simulink model "SOC_Estimation_2RC"  (R2022a)
settings: Solver=VariableStepAuto  StartTime=0.0  StopTime=3600  RelTol=1e-3
libraries: fl_lib x9, nesl_utility x4, simulink x2
settings Model: Creator=10109  LastModifiedBy=10109

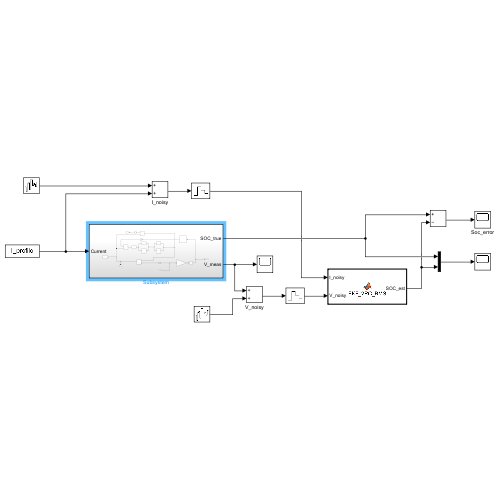
[thumbnail: Simulink's stored preview of the top-level diagram]
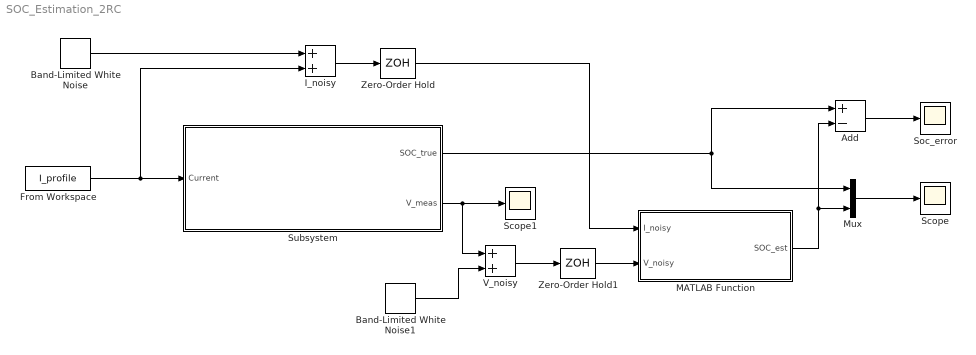
== system SOC_Estimation_2RC ==
  Add : Sum  Inputs=+-
  Band-Limited White Noise : simulink/Sources/Band-Limited White Noise  Cov=[4e-4]  Ts=1  seed=[2334]
  Band-Limited White Noise1 : simulink/Sources/Band-Limited White Noise  Cov=[1e-4]  Ts=1  seed=[2335]
  From Workspace : FromWorkspace  VariableName=I_profile
  I_noisy : Sum
  MATLAB Function : MATLAB Function  TreatAsAtomicUnit=on
  Mux : Mux  Inputs=2
  Scope : Scope
  Scope1 : Scope
  Soc_error : Scope
  Subsystem : Subsystem
  V_noisy : Sum
  Zero-Order Hold : ZeroOrderHold
  Zero-Order Hold1 : ZeroOrderHold
  wires:
  Subsystem/2(V_meas) -> Scope1/1, V_noisy/1
  Band-Limited White Noise1/1 -> V_noisy/2
  From Workspace/1 -> Subsystem/1(Current), I_noisy/2
  Band-Limited White Noise/1 -> I_noisy/1
  Subsystem/1(SOC_true) -> Add/1, Mux/1
  MATLAB Function/1(SOC_est) -> Add/2, Mux/2
  Zero-Order Hold1/1 -> MATLAB Function/2(V_noisy)
  I_noisy/1 -> Zero-Order Hold/1
  Zero-Order Hold/1 -> MATLAB Function/1(I_noisy)
  V_noisy/1 -> Zero-Order Hold1/1
  Mux/1 -> Scope/1
  Add/1 -> Soc_error/1

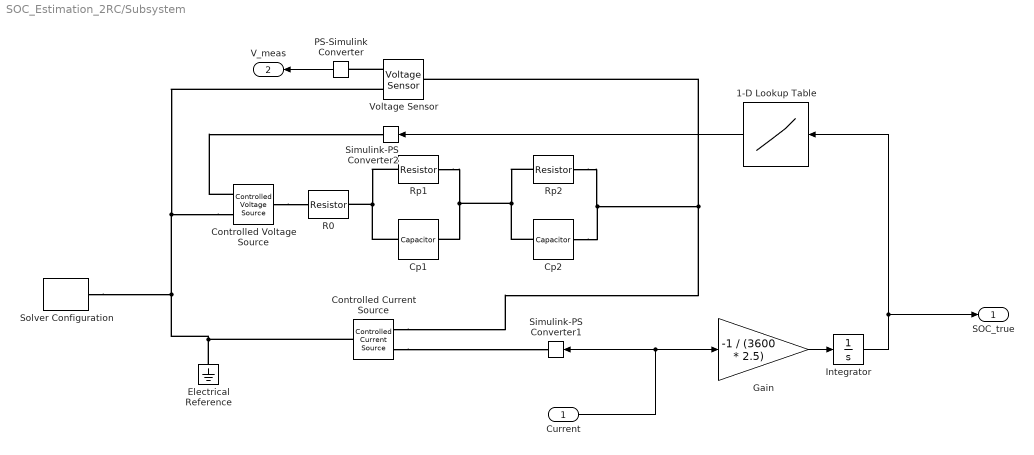
== system SOC_Estimation_2RC/Subsystem ==
  Current : Inport
  1-D Lookup Table : Lookup_n-D  NumberOfTableDimensions=1  BreakpointsForDimension1=[0, 0.1, 0.2, 0.3, 0.4, 0.5, 0.6, 0.7, 0.8, 0.9, 1.0]  Table=[3.00, 3.45, 3.55, 3.62, 3.68, 3.74, 3.82, 3.92, 4.02, 4.12, 4.20]  ExtrapMethod=Clip  UseLastTableValue=on  InternalRulePriority=Speed  RndMeth=Simplest
  Controlled Current Source : fl_lib/Electrical/Electrical Sources/Controlled Current Source
      settings: SourceProductBaseCode=PW,SS,VE
  Controlled Voltage Source : fl_lib/Electrical/Electrical Sources/Controlled Voltage Source
      settings: SourceProductBaseCode=PW,SS,VE
  Cp1 : fl_lib/Electrical/Electrical Elements/Capacitor  c=250 F  r=1e-6 Ohm  g=0 1/Ohm  i_specify=off  i_priority=None  i=0 A  i_nominal_specify=off  i_nominal_unit=A  i_nominal_value=1  v_specify=off  v_priority=None  v=0 V  v_nominal_specify=off  v_nominal_unit=V  v_nominal_value=1  vc_specify=off  vc_priority=High  vc=0 V  vc_nominal_specify=off  vc_nominal_unit=V  vc_nominal_value=1
      settings: SourceProductBaseCode=PW,SS,VE
  Cp2 : fl_lib/Electrical/Electrical Elements/Capacitor  c=1200 F  r=1e-6 Ohm  g=0 1/Ohm  i_specify=off  i_priority=None  i=0 A  i_nominal_specify=off  i_nominal_unit=A  i_nominal_value=1  v_specify=off  v_priority=None  v=0 V  v_nominal_specify=off  v_nominal_unit=V  v_nominal_value=1  vc_specify=off  vc_priority=High  vc=0 V  vc_nominal_specify=off  vc_nominal_unit=V  vc_nominal_value=1
      settings: SourceProductBaseCode=PW,SS,VE
  Electrical Reference : fl_lib/Electrical/Electrical Elements/Electrical Reference
      settings: SourceProductBaseCode=PW,SS,VE
  Gain : Gain  Gain=-1 / (3600 * 2.5)
  Integrator : Integrator  InitialCondition=1.0
  PS-Simulink Converter : nesl_utility/PS-Simulink Converter  PhysicalDomain=network_engine_domain  SubClassName=ps_output  LeftPortType=input  RightPortType=output  PseudoPeriodic=off  Frequencies=[]  VectorFormat=inherit  Unit=inherit  AffineConversion=off
      settings: SourceProductBaseCode=SS,PW,VE
  R0 : fl_lib/Electrical/Electrical Elements/Resistor  R=0.025 Ohm  i_specify=off  i_priority=None  i=0 A  i_nominal_specify=off  i_nominal_unit=A  i_nominal_value=1  v_specify=off  v_priority=None  v=0 V  v_nominal_specify=off  v_nominal_unit=V  v_nominal_value=1
      settings: SourceProductBaseCode=PW,SS,VE
  Rp1 : fl_lib/Electrical/Electrical Elements/Resistor  R=0.01 Ohm  i_specify=off  i_priority=None  i=0 A  i_nominal_specify=off  i_nominal_unit=A  i_nominal_value=1  v_specify=off  v_priority=None  v=0 V  v_nominal_specify=off  v_nominal_unit=V  v_nominal_value=1
      settings: SourceProductBaseCode=PW,SS,VE
  Rp2 : fl_lib/Electrical/Electrical Elements/Resistor  R=0.015 Ohm  i_specify=off  i_priority=None  i=0 A  i_nominal_specify=off  i_nominal_unit=A  i_nominal_value=1  v_specify=off  v_priority=None  v=0 V  v_nominal_specify=off  v_nominal_unit=V  v_nominal_value=1
      settings: SourceProductBaseCode=PW,SS,VE
  Simulink-PS Converter1 : nesl_utility/Simulink-PS Converter  PhysicalDomain=network_engine_domain  SubClassName=ps_input  LeftPortType=input  RightPortType=output  PseudoPeriodic=off  Frequencies=[]  NoiseDistribution=none  NoiseParameters=[]  Unit=1  AffineConversion=off  FilteringAndDerivatives=provide  SimscapeFilterOrder=1  InputFilterTimeConstant=0.001  UdotUserProvided=0
      settings: SourceProductBaseCode=SS,PW,VE
  Simulink-PS Converter2 : nesl_utility/Simulink-PS Converter  PhysicalDomain=network_engine_domain  SubClassName=ps_input  LeftPortType=input  RightPortType=output  PseudoPeriodic=off  Frequencies=[]  NoiseDistribution=none  NoiseParameters=[]  Unit=1  AffineConversion=off  FilteringAndDerivatives=provide  SimscapeFilterOrder=1  InputFilterTimeConstant=0.001  UdotUserProvided=0
      settings: SourceProductBaseCode=SS,PW,VE
  Solver Configuration : nesl_utility/Solver Configuration  PhysicalDomain=network_engine_domain  SubClassName=solver  LeftPortType=input  RightPortType=generic  Tones=[]  Harmonics=[]  SimulateNoise=off  Profile=off  UseLocalSampling=off  EnableSwitchedLinearOptims=on  FrequencyDomain=off  UseCCode=off  RelTol=0.001  AbsTol=0.001  MinStep=1e-09  ToWorkspace=off  RevertToSquareIcSolve=off  NumHomotopyIterations=100  PhasorMode=off  PhasorModeNumHarmonics=1  IndexReductionMethod=DerivativeReplacement  DoDC=off  ResidualTolerance=1e-09  UseLocalSolver=off  LocalSolverChoice=NE_BACKWARD_EULER_ADVANCER  LocalSolverSampleTime=0.001  DoFixedCost=off  MaxNonlinIter=3  MaxModeIter=2  ComputeImpulses=off  ImpulseIterations=2  LinearAlgebra=auto  LinearAlgebraNumThread=0  EquationFormulation=NE_TIME_EF  DelaysMemoryBudget=1024  AutomaticFiltering=on  FilteringTimeConstant=0.001  PartitionStorageMethod=AS_NEEDED  PartitionMemoryBudget=1024  PartitionMethod=ROBUST
      settings: SourceProductBaseCode=SS,PW,VE
  Voltage Sensor : fl_lib/Electrical/Electrical Sensors/Voltage Sensor
      settings: SourceProductBaseCode=PW,SS,VE
  SOC_true : Outport
  V_meas : Outport  Port=2
  wires:
  Current/1 -> Simulink-PS Converter1/1, Gain/1
  Integrator/1 -> SOC_true/1, 1-D Lookup Table/1
  PS-Simulink Converter/1 -> V_meas/1
  Gain/1 -> Integrator/1
  1-D Lookup Table/1 -> Simulink-PS Converter2/1
  connections:
  Controlled Voltage Source/RConn2 -- Controlled Current Source/LConn1 -- Electrical Reference/LConn1 -- Solver Configuration/RConn1 -- Voltage Sensor/RConn2
  Rp2/RConn1 -- Cp2/RConn1 -- Voltage Sensor/LConn1 -- Controlled Current Source/RConn2
  R0/RConn1 -- Cp1/LConn1 -- Rp1/LConn1
  Voltage Sensor/RConn1 -- PS-Simulink Converter/LConn1
  Controlled Voltage Source/LConn1 -- R0/LConn1
  Rp1/RConn1 -- Rp2/LConn1 -- Cp2/LConn1 -- Cp1/RConn1
  Controlled Current Source/RConn1 -- Simulink-PS Converter1/RConn1
  Controlled Voltage Source/RConn1 -- Simulink-PS Converter2/RConn1

== matlab function SOC_Estimation_2RC/MATLAB Function ==
  data: I_noisy input; SOC_est output; V_noisy input
function SOC_est = EKF_2RC_BMS(I_noisy, V_noisy)
%% 1. 真实三元锂 (NMC) 2RC 模型参数
    R0 = 0.025;      
    Rp1 = 0.010;  Cp1 = 250;   % 快响应极化
    Rp2 = 0.015;  Cp2 = 1200;  % 慢响应极化
    Cn = 2.5 * 3600;           % 容量 (As)
    dt = 1;                    % 步长 (s)
    
    soc_table = [0, 0.1, 0.2, 0.3, 0.4, 0.5, 0.6, 0.7, 0.8, 0.9, 1.0];
    ocv_table = [3.00, 3.45, 3.55, 3.62, 3.68, 3.74, 3.82, 3.92, 4.02, 4.12, 4.20];

    %% 2. 状态与协方差初始化 (扩维到 3x3)
    persistent x_hat P
    if isempty(x_hat)
        x_hat = [0.8; 0; 0]; % 初始猜测: SOC=0.8, Up1=0, Up2=0
        P = diag([1e-4, 1e-4, 1e-4]); 
    end
    
    %% 3. 噪声协方差矩阵 (Q 扩维到 3x3)
    Q = diag([1e-6, 1e-5, 1e-5]); 
    R_cov = 1e-2;                 

    %% ================= EKF 核心五步 (3阶矩阵运算) ================= %%
    
    % 时间常数计算
    tau1 = Rp1 * Cp1;
    tau2 = Rp2 * Cp2;

    % 【步骤一：状态预测】离散化 A 和 B 矩阵
    A = [1, 0, 0; 
         0, exp(-dt/tau1), 0;
         0, 0, exp(-dt/tau2)];
         
    B = [-dt/Cn; 
         Rp1*(1 - exp(-dt/tau1));
         Rp2*(1 - exp(-dt/tau2))];
     
    x_pred = A * x_hat + B * I_noisy;
    
    % 限制 SOC 边界防报错
    soc_pred = x_pred(1);
    if soc_pred > 1, soc_pred = 1; end
    if soc_pred < 0, soc_pred = 0; end
    
    % 【步骤二：协方差预测】
    P_pred = A * P * A' + Q;
    
    % 【步骤三：雅可比矩阵 H】
    delta_soc = 0.01;
    ocv_plus = interp1(soc_table, ocv_table, min(1, soc_pred + delta_soc), 'linear', 'extrap');
    ocv_minus = interp1(soc_table, ocv_table, max(0, soc_pred - delta_soc), 'linear', 'extrap');
    dOCV_dSOC = (ocv_plus - ocv_minus) / (2 * delta_soc);
    
    % H 矩阵扩维: [dOCV/dSOC, -1, -1]
    H = [dOCV_dSOC, -1, -1];
    
    % 预测端电压 V_pred = OCV - Up1 - Up2 - I*R0
    OCV_pred = interp1(soc_table, ocv_table, soc_pred, 'linear', 'extrap');
    V_pred = OCV_pred - x_pred(2) - x_pred(3) - I_noisy * R0;
    
    % 【步骤四：计算卡尔曼增益 K】
    K = P_pred * H' / (H * P_pred * H' + R_cov);
    
    % 【步骤五：状态与协方差更新】
    x_hat = x_pred + K * (V_noisy - V_pred);
    P = (eye(3) - K * H) * P_pred;
    
    %% 4. 输出
    SOC_est = x_hat(1);
end
